simulink model "LowPassFilter2p2"  (R2019b)
settings: Solver=ode1  StartTime=0.0  StopTime=10  FixedStep=Tn  RelTol=1e-3
values from neighbouring files (symbols this model uses):
  curr_freq = 2    [LowPassFilter2_pram.m]
  sample_freq = 1/Tn    (= 1000)    [LowPassFilter2_pram.m]
  Tn = 0.001    [LowPassFilter2_pram.m]
  wn = curr_freq*pi*2    (= 12.5663706144)    [LowPassFilter2_pram.m]
  zuni = cos(pi/4.0)    [LowPassFilter2_pram.m]
settings Model: Creator=a4327  LastModifiedBy=a4327
settings OptimizationCC: DefaultParameterBehavior=Inlined  UseDivisionForNetSlopeComputation=on  GainParamInheritBuiltInType=on  UseFloatMulNetSlope=on  InlineInvariantSignals=on  PassReuseOutputArgsAs=Individual arguments  ZeroExternalMemoryAtStartup=off  ZeroInternalMemoryAtStartup=off  NoFixptDivByZeroProtection=on  EfficientFloat2IntCast=on  LifeSpan=1  OptimizeBlockOrder=speed  DifferentSizesBufferReuse=on  EfficientTunableParamExpr=on
settings DebuggingCC: ParameterTunabilityLossMsg=error
settings HardwareCC: ProdBitPerPointer=32  ProdBitPerSizeT=32  ProdBitPerPtrDiffT=32  ProdLargestAtomicFloat=None  ProdWordSize=32  ProdLongLongMode=on  ProdHWDeviceType=Custom Processor->Custom Processor
settings SFSimCC: MATLABDynamicMemAlloc=off
settings RTWCC: SystemTargetFile=ert.tlc  TemplateMakefile=ert_default_tmf  GenerateReport=on  IncludeHyperlinkInReport=on  LaunchReport=on  GenerateTraceInfo=on  GenerateTraceReport=on  GenerateTraceReportSl=on  GenerateTraceReportSf=on  GenerateTraceReportEml=on  GenerateCodeMetricsReport=on
settings CodeAppCC: ForceParamTrailComments=on  IgnoreCustomStorageClasses=off  OperatorAnnotations=on  SimulinkDataObjDesc=on  SFDataObjDesc=on  CustomSymbolStrGlobalVar=rt$N$M  CustomSymbolStrType=$N$M  CustomSymbolStrFcn=$N$M$F  CustomSymbolStrMacro=$N$M  InsertBlockDesc=on
settings ERTTargetCC: TargetLangStandard=C99 (ISO)  GenerateSampleERTMain=on  IncludeMdlTerminateFcn=off  CombineSignalStateStructs=on  SupportComplex=off  SupportNonInlinedSFcns=on  InlinedParameterPlacement=NonHierarchical  ERTCustomFileTemplate=example_file_process.tlc  ERTFilePackagingFormat=CompactWithDataFile

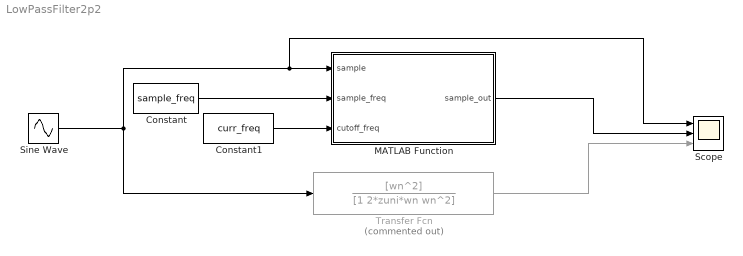
== system LowPassFilter2p2 ==
  Constant : Constant  Value=sample_freq
  Constant1 : Constant  Value=curr_freq
  MATLAB Function : MATLAB Function  TreatAsAtomicUnit=on
  Scope : Scope  NumInputPorts=3
  Sine Wave : Sin  Frequency=2*pi*2  SampleTime=Tn
  Transfer Fcn : TransferFcn  Commented=on  Numerator=[wn^2]  Denominator=[1 2*zuni*wn wn^2]
  wires:
  Constant/1 -> MATLAB Function/2(sample_freq)
  Constant1/1 -> MATLAB Function/3(cutoff_freq)
  Sine Wave/1 -> Scope/1, MATLAB Function/1(sample), Transfer Fcn/1
  Transfer Fcn/1 -> Scope/3
  MATLAB Function/1(sample_out) -> Scope/2

== matlab function LowPassFilter2p2/MATLAB Function ==
  data: sample input; sample_out output; sample_freq input; cutoff_freq input
function sample_out = LowPassFilter2p(sample,sample_freq,  cutoff_freq)

persistent params
    if isempty(params)
    params=compute_params( sample_freq,  cutoff_freq);
    end
sample_out= DigitalBiquadFilter_apply(sample, params);
